simulink model "homework1"  (R2024b)
settings: Solver=ode1  StartTime=0.0  StopTime=100.0  FixedStep=0.001  RelTol=1e-3
settings Model: Creator=eitherwoods  LastModifiedBy=eitherwoods

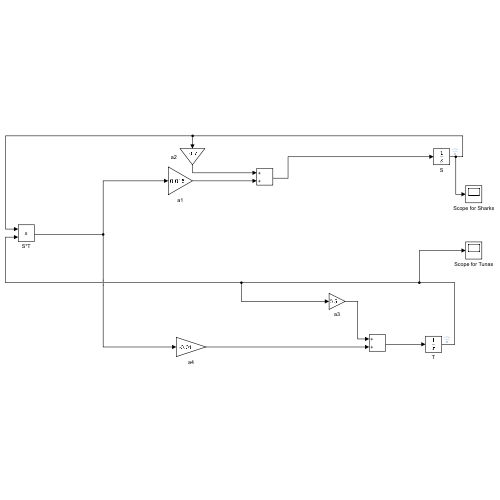
[thumbnail: Simulink's stored preview of the top-level diagram]
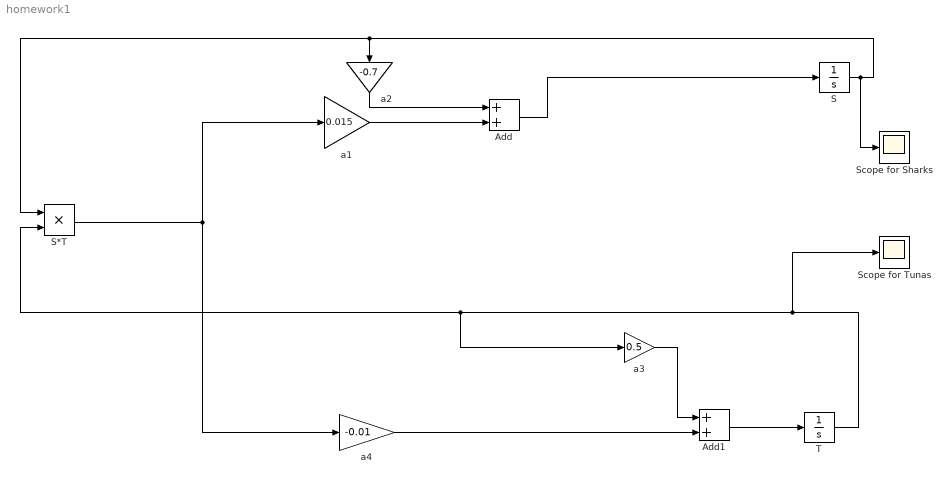
== system homework1 ==
  Add : Sum
  Add1 : Sum
  S : Integrator  InitialCondition=100
  S*T : Product
  Scope for Sharks : Scope
  Scope for Tunas : Scope
  T : Integrator  InitialCondition=100
  a1 : Gain  Gain=0.015
  a2 : Gain  Gain=-0.7
  a3 : Gain  Gain=0.5
  a4 : Gain  Gain=-0.01
  wires:
  S/1 -> Scope for Sharks/1, S*T/1, a2/1
  T/1 -> Scope for Tunas/1, a3/1, S*T/2
  S*T/1 -> a4/1, a1/1
  a1/1 -> Add/2
  a2/1 -> Add/1
  Add/1 -> S/1
  a4/1 -> Add1/2
  a3/1 -> Add1/1
  Add1/1 -> T/1
